simulink model "Upper_Humanoid"  (R2023a)
settings: Solver=VariableStepAuto  StartTime=0.0  StopTime=10  RelTol=1e-3
undefined symbols (not defined in the file or in its folder): smiData, smiData1, X, Y, Z
libraries: sm_lib x268, nesl_utility x32, simulink_extras x8
(part 6 of 6)

== matlab function Upper_Humanoid/MATLAB Function5 ==
  data: X_r input; q output; q0 input
function q   = Rob_inverseandforward_kinematics(X_r,q0)
    l1 = 0.0288811487749;%old: 0.0291
    l2 = 0.02659997;%old: 0.04406
    l3 = 0.12240002;%old: 0.10416
    l4 = 0.15;%old: 0.15444
    x=0;
    y=0;
    z=0;
    J = zeros(3,4);
    %Calculate the inverse Jacobian matrix
    
    q = q0 ;
    maxError = 10^-8;
    error = inf;
     % 
     while error > maxError
            
            q1 = q(1,1);
            q2 = q(2,1);
            q3 = q(3,1);
            q4 = q(4,1);
            
          
    
    X = [l4*cos((pi*q1)/180)*sin((pi*(q2 - 90))/180)*sin((pi*(q4 - 90))/180)-l4*cos((pi*(q4 - 90))/180)*(sin((pi*q1)/180)*sin((pi*(q3 - 90))/180)-cos((pi*q1)/180)*cos((pi*(q2 - 90))/180)*cos((pi*(q3 - 90))/180))-cos((pi*q1)/180)*sin((pi*(q2 - 90))/180)*(l2 + l3);
        l4*cos((pi*(q4 - 90))/180)*(cos((pi*q1)/180)*sin((pi*(q3 - 90))/180)+sin((pi*q1)/180)*cos((pi*(q2 - 90))/180)*cos((pi*(q3 - 90))/180))-sin((pi*q1)/180)*sin((pi*(q2 - 90))/180)*(l2 + l3)+l4*sin((pi*q1)/180)*sin((pi*(q2 - 90))/180)*sin((pi*(q4 - 90))/180);
        l4*cos((pi*(q2 - 90))/180)*sin((pi*(q4 - 90))/180)-cos((pi*(q2 - 90))/180)*(l2 + l3)-l1-l4*cos((pi*(q3 - 90))/180)*cos((pi*(q4 - 90))/180)*sin((pi*(q2 - 90))/180)];
 
    x = X(1,1);
    y = X(2,1);
    z = X(3,1);
           
    
            x_current = [x;y;z];
             
           
            % if error < maxError
            %     break;
            % end
     
            Jac= [(l4*pi*sin((pi*q4)/180)*(cos((pi*q1)/180)*cos((pi*q3)/180)-sin((pi*q1)/180)*sin((pi*q2)/180)*sin((pi*q3)/180)))/180 - (pi*cos((pi*q2)/180)*sin((pi*q1)/180)*(l2 + l3))/180 - (l4*pi*cos((pi*q2)/180)*cos((pi*q4)/180)*sin((pi*q1)/180))/180,                          -(pi*cos((pi*q1)/180)*(l2*sin((pi*q2)/180) + l3*sin((pi*q2)/180) + l4*cos((pi*q4)/180)*sin((pi*q2)/180) - l4*cos((pi*q2)/180)*sin((pi*q3)/180)*sin((pi*q4)/180)))/180, -(l4*pi*sin((pi*q4)/180)*(sin((pi*q1)/180)*sin((pi*q3)/180) - cos((pi*q1)/180)*cos((pi*q3)/180)*sin((pi*q2)/180)))/180,   (l4*pi*cos((pi*q4)/180)*(cos((pi*q3)/180)*sin((pi*q1)/180) + cos((pi*q1)/180)*sin((pi*q2)/180)*sin((pi*q3)/180)))/180 - (l4*pi*cos((pi*q1)/180)*cos((pi*q2)/180)*sin((pi*q4)/180))/180;
                 (l4*pi*sin((pi*q4)/180)*(cos((pi*q3)/180)*sin((pi*q1)/180)+ cos((pi*q1)/180)*sin((pi*q2)/180)*sin((pi*q3)/180)))/180 + (pi*cos((pi*q1)/180)*cos((pi*q2)/180)*(l2 + l3))/180 + (l4*pi*cos((pi*q1)/180)*cos((pi*q2)/180)*cos((pi*q4)/180))/180,                          -(pi*sin((pi*q1)/180)*(l2*sin((pi*q2)/180) + l3*sin((pi*q2)/180) + l4*cos((pi*q4)/180)*sin((pi*q2)/180) - l4*cos((pi*q2)/180)*sin((pi*q3)/180)*sin((pi*q4)/180)))/180,  (l4*pi*sin((pi*q4)/180)*(cos((pi*q1)/180)*sin((pi*q3)/180) + cos((pi*q3)/180)*sin((pi*q1)/180)*sin((pi*q2)/180)))/180, - (l4*pi*cos((pi*q4)/180)*(cos((pi*q1)/180)*cos((pi*q3)/180) - sin((pi*q1)/180)*sin((pi*q2)/180)*sin((pi*q3)/180)))/180 - (l4*pi*cos((pi*q2)/180)*sin((pi*q1)/180)*sin((pi*q4)/180))/180;
                                                                                                                                                                                                                                                      0, (pi*sin((pi*(q2 - 90))/180)*(l2 + l3))/180 - (l4*pi*sin((pi*(q2 - 90))/180)*sin((pi*(q4 - 90))/180))/180 - (l4*pi*cos((pi*(q2 - 90))/180)*cos((pi*(q3 - 90))/180)*cos((pi*(q4 - 90))/180))/180,                                                         (l4*pi*cos((pi*q2)/180)*cos((pi*q3)/180)*sin((pi*q4)/180))/180,                                                                           (l4*pi*sin((pi*q2)/180)*sin((pi*q4)/180))/180 + (l4*pi*cos((pi*q2)/180)*cos((pi*q4)/180)*sin((pi*q3)/180))/180;
                                                                                                                                                                                                                                                            0,                                                                                                                                                                        sin((pi*(q2 - 90))/180),                                                                                     -cos((pi*q3)/180)*sin((pi*q2)/180),                                                                                                                                                       -cos((pi*q3)/180)*sin((pi*q2)/180);
                                                                                                                                                                                                                                                      0,                                                                                                                                                                       -cos((pi*(q2 - 90))/180),                                                                                      cos((pi*q2)/180)*cos((pi*q3)/180),                                                                                                                                                        cos((pi*q2)/180)*cos((pi*q3)/180);
                                                                                                                                                                                                                                                       1,                                                                                                                                                                                              0,                                                                                               -cos((pi*(q3 - 90))/180),                                                                                                                                                                 -cos((pi*(q3 - 90))/180)]
            J = Jac(1:3,:);  
            fakeJ =pinv(J);
            x_error =  x_current-X_r;
            q = (double(q - fakeJ* x_error));
            % q=wrapToPi(q)
            error = norm(x_error);
          
        
        end

== matlab function Upper_Humanoid/MATLAB Function ==
  data: X0 input; out1 output; Xf input; Tf input; t input; out2 output
function [out1,out2] = tasktraj(X0, Xf, Tf, t)

x0=X0(1);
y0=X0(2);
z0=X0(3);
xf=Xf(1);
yf=Xf(2);
zf=Xf(3);
Tf1 = (Tf/3);
Tf2= 2*(Tf/3);
%Task_Space = [];
if(t<Tf1)
x = x0 + ((xf-x0)/Tf1)*t;
y = y0 ;
z = z0 ;
else
    if t<Tf2
    x =Xf(1);
    z=z0
    y = y0 + ((yf-y0)/Tf1)*(t-Tf1);
    else
    z = z0 + ((zf-z0)/Tf1)*(t-Tf2);
    x =Xf(1);
    y=Xf(2)
    end
end
out1=[x;y;z];
out2=[x;y;-z];

== matlab function Upper_Humanoid/MATLAB Function1 ==
  data: X_r input; q output; q0 input
function q   = Rob_inverseandforward_kinematics(X_r,q0)
    l1 = 0.0288811487749;%old: 0.0291
    l2 = 0.02659997;%old: 0.04406
    l3 = 0.12240002;%old: 0.10416
    l4 = 0.15;%old: 0.15444
    x=0;
    y=0;
    z=0;
    J = zeros(3,4);
    %Calculate the inverse Jacobian matrix
    
    q = q0 ;
    maxError = 10^-8;
    error = inf;
     % 
     while error > maxError
            
            Q1 = q(1,1);
            Q2 = q(2,1);
            Q3 = q(3,1);
            Q4 = q(4,1);
            
          
    
    X = [ 
(19*cos((pi*Q1)/180)*sin((pi*(Q2 - 90))/180)*sin((pi*(Q4 - 90))/180))/125 - (1093*cos((pi*Q1)/180)*sin((pi*(Q2 - 90))/180))/10000 - (19*cos((pi*(Q4 - 90))/180)*(sin((pi*Q1)/180)*sin((pi*(Q3 - 90))/180) - cos((pi*Q1)/180)*cos((pi*(Q2 - 90))/180)*cos((pi*(Q3 - 90))/180)))/125;
(19*cos((pi*(Q4 - 90))/180)*(cos((pi*Q1)/180)*sin((pi*(Q3 - 90))/180) + sin((pi*Q1)/180)*cos((pi*(Q2 - 90))/180)*cos((pi*(Q3 - 90))/180)))/125 - (1093*sin((pi*Q1)/180)*sin((pi*(Q2 - 90))/180))/10000 + (19*sin((pi*Q1)/180)*sin((pi*(Q2 - 90))/180)*sin((pi*(Q4 - 90))/180))/125;
                                                                                      (1093*cos((pi*(Q2 - 90))/180))/10000 - (19*cos((pi*(Q2 - 90))/180)*sin((pi*(Q4 - 90))/180))/125 + (19*cos((pi*(Q3 - 90))/180)*cos((pi*(Q4 - 90))/180)*sin((pi*(Q2 - 90))/180))/125 + 81/2500];
 
    x = X(1,1);
    y = X(2,1);
    z = X(3,1);
           
    
            x_current = [x;y;z];
             
           
            % if error < maxError
            %     break;
            % end
     
            J= [(19*pi*sin((pi*Q4)/180)*(cos((pi*Q1)/180)*cos((pi*Q3)/180) - sin((pi*Q1)/180)*sin((pi*Q2)/180)*sin((pi*Q3)/180)))/22500 - (1093*pi*cos((pi*Q2)/180)*sin((pi*Q1)/180))/1800000 - (19*pi*cos((pi*Q2)/180)*cos((pi*Q4)/180)*sin((pi*Q1)/180))/22500, -(pi*cos((pi*Q1)/180)*(1093*sin((pi*Q2)/180) + 1520*cos((pi*Q4)/180)*sin((pi*Q2)/180) - 1520*cos((pi*Q2)/180)*sin((pi*Q3)/180)*sin((pi*Q4)/180)))/1800000, -(19*pi*sin((pi*Q4)/180)*(sin((pi*Q1)/180)*sin((pi*Q3)/180) - cos((pi*Q1)/180)*cos((pi*Q3)/180)*sin((pi*Q2)/180)))/22500,   (19*pi*cos((pi*Q4)/180)*(cos((pi*Q3)/180)*sin((pi*Q1)/180) + cos((pi*Q1)/180)*sin((pi*Q2)/180)*sin((pi*Q3)/180)))/22500 - (19*pi*cos((pi*Q1)/180)*cos((pi*Q2)/180)*sin((pi*Q4)/180))/22500;
(19*pi*sin((pi*Q4)/180)*(cos((pi*Q3)/180)*sin((pi*Q1)/180) + cos((pi*Q1)/180)*sin((pi*Q2)/180)*sin((pi*Q3)/180)))/22500 + (1093*pi*cos((pi*Q1)/180)*cos((pi*Q2)/180))/1800000 + (19*pi*cos((pi*Q1)/180)*cos((pi*Q2)/180)*cos((pi*Q4)/180))/22500, -(pi*sin((pi*Q1)/180)*(1093*sin((pi*Q2)/180) + 1520*cos((pi*Q4)/180)*sin((pi*Q2)/180) - 1520*cos((pi*Q2)/180)*sin((pi*Q3)/180)*sin((pi*Q4)/180)))/1800000,  (19*pi*sin((pi*Q4)/180)*(cos((pi*Q1)/180)*sin((pi*Q3)/180) + cos((pi*Q3)/180)*sin((pi*Q1)/180)*sin((pi*Q2)/180)))/22500, - (19*pi*cos((pi*Q4)/180)*(cos((pi*Q1)/180)*cos((pi*Q3)/180) - sin((pi*Q1)/180)*sin((pi*Q2)/180)*sin((pi*Q3)/180)))/22500 - (19*pi*cos((pi*Q2)/180)*sin((pi*Q1)/180)*sin((pi*Q4)/180))/22500;
                                                                                                                                                                                                                                               0,   (1093*pi*cos((pi*Q2)/180))/1800000 + (19*pi*cos((pi*Q2)/180)*cos((pi*Q4)/180))/22500 + (19*pi*sin((pi*Q2)/180)*sin((pi*Q3)/180)*sin((pi*Q4)/180))/22500,                                                        -(19*pi*cos((pi*Q2)/180)*cos((pi*Q3)/180)*sin((pi*Q4)/180))/22500,                                                                         - (19*pi*sin((pi*Q2)/180)*sin((pi*Q4)/180))/22500 - (19*pi*cos((pi*Q2)/180)*cos((pi*Q4)/180)*sin((pi*Q3)/180))/22500];

            fakeJ =pinv(J);
            x_error =  x_current-X_r;
            q = (double(q - fakeJ* x_error));
            % q=wrapToPi(q)
            error = norm(x_error);
          
        
        end
